simulink model "carSusSim"  (R2024b)
settings: Solver=VariableStepAuto  StartTime=0.0  StopTime=10.0  RelTol=1e-3
values from neighbouring files (symbols this model uses):
  carSusTF = tf(carSusSS)    [carSus.m]
settings Model: Creator=steve0gillet  LastModifiedBy=steve0gillet
settings DataIOCC: ReturnWorkspaceOutputs=off

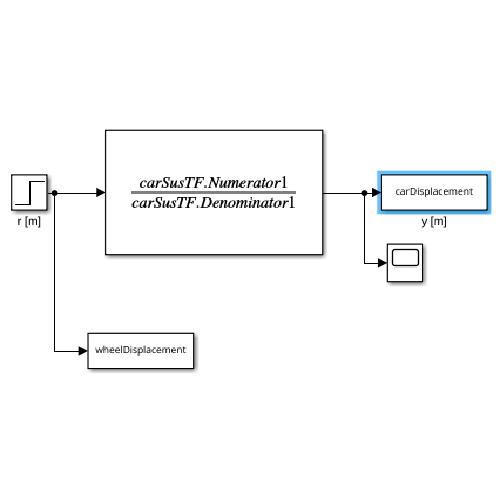
[thumbnail: Simulink's stored preview of the top-level diagram]
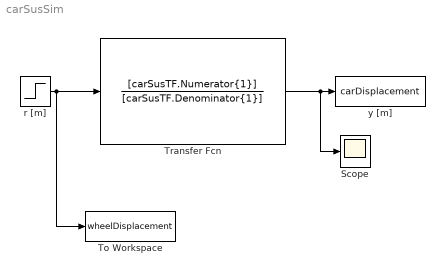
== system carSusSim ==
  Scope : Scope
  To Workspace : ToWorkspace  VariableName=wheelDisplacement  SaveFormat=Timeseries  SampleTime=-1
  Transfer Fcn : TransferFcn  Numerator=[carSusTF.Numerator{1}]  Denominator=[carSusTF.Denominator{1}]
  r [m] : Step  SampleTime=0
  y [m] : ToWorkspace  VariableName=carDisplacement  SaveFormat=Timeseries  SampleTime=-1
  wires:
  r [m]/1 -> To Workspace/1, Transfer Fcn/1
  Transfer Fcn/1 -> Scope/1, y [m]/1
